simulink subsystem "Tester_subsystem"  (R2023b)
settings: Solver=VariableStepAuto  StartTime=0.0  StopTime=10.0  RelTol=1e-3
settings Model: Creator=nickj  LastModifiedBy=diego

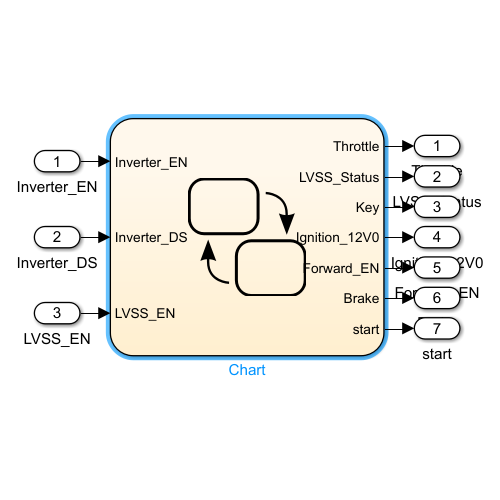
[thumbnail: Simulink's stored preview of the top-level diagram]
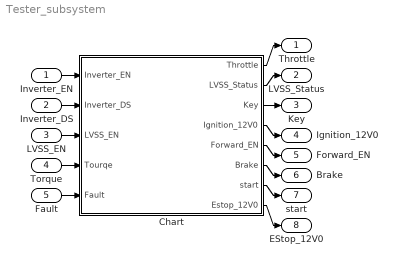
== system Tester_subsystem ==
  Inverter_EN : Inport
  Inverter_DS : Inport  Port=2
  LVSS_EN : Inport  Port=3
  Torque : Inport  Port=4
  Fault : Inport  Port=5
  Chart : Stateflow chart  TreatAsAtomicUnit=on
  Throttle : Outport
  LVSS_Status : Outport  Port=2
  Key : Outport  Port=3
  Ignition_12V0 : Outport  Port=4
  Forward_EN : Outport  Port=5
  Brake : Outport  Port=6
  start : Outport  Port=7
  EStop_12V0 : Outport  Port=8
  wires:
  Chart/3(Key) -> Key/1
  Chart/7(start) -> start/1
  Chart/6(Brake) -> Brake/1
  Chart/1(Throttle) -> Throttle/1
  Inverter_EN/1 -> Chart/1(Inverter_EN)
  Inverter_DS/1 -> Chart/2(Inverter_DS)
  LVSS_EN/1 -> Chart/3(LVSS_EN)
  Chart/4(Ignition_12V0) -> Ignition_12V0/1
  Chart/2(LVSS_Status) -> LVSS_Status/1
  Chart/5(Forward_EN) -> Forward_EN/1
  Torque/1 -> Chart/4(Tourqe)
  Fault/1 -> Chart/5(Fault)
  Chart/8(Estop_12V0) -> EStop_12V0/1

== stateflow chart Tester_subsystem/Chart ==
  state Test_proc
    state Key_Proc
      entry:
      Key = 1;
      Ignition_12V0 = 1;
    state LVSS_Start_Proc
      entry:
      LVSS_Status = 1;
    state Contactor_Closed_Proc
      entry:
      Forward_EN = 1;
      Brake = 1;
      Throttle = 0;
      start = 1;
    state Contactor_Closed_Proc_2
      entry:
      Forward_EN = 1;
      Brake = 1;
      Throttle = 0;
      start = 1;
    state MC_Active_Proc
      entry:
      Forward_EN = 0;
    state MC_Active_Proc1
      entry:
      Ignition_12V0 = 0;
    state LVSS_Shutdown_Proc
      entry:
      LVSS_Status = 0;
    state Off_Proc2
      entry:
      Key = 1;
      Ignition_12V0 = 1;
      LVSS_Status = 1;
    state Init_Proc
      entry:
      Ignition_12V0 = 0;
      LVSS_Status = 0;
    state Off_Proc
      entry:
      Key = 1;
      Ignition_12V0 = 1;
      LVSS_Status = 1;
    state Off_Estop_Proc
      entry:
      Key = 1;
      Ignition_12V0 = 1;
      LVSS_Status = 1;
    state Estop_Proc
      entry:
      Estop_12V0 = 1;
    (default) -> Key_Proc
    Key_Proc -> LVSS_Start_Proc : [LVSS_EN == 1 && Fault == 0]
    Test_proc -> Key_Proc : [LVSS_EN ==0 && Inverter_DS == 1]
    LVSS_Start_Proc -> Contactor_Closed_Proc : [Inverter_DS == 1 && Fault == 0]
    Contactor_Closed_Proc -> MC_Active_Proc : [Inverter_EN == 1 && Tourqe == 0 && Fault == 0]
    MC_Active_Proc -> Contactor_Closed_Proc_2 : [Inverter_EN == 0 && Fault == 0]
    Contactor_Closed_Proc_2 -> MC_Active_Proc1 : [Inverter_EN == 1 && Fault == 0]
    MC_Active_Proc1 -> LVSS_Shutdown_Proc : [Inverter_EN == 0 && Inverter_DS == 1 && Fault == 0]
    LVSS_Shutdown_Proc -> Off_Proc : [LVSS_EN == 0 && Inverter_EN == 0 && Fault == 0]
    Init_Proc -> Off_Proc2 : [LVSS_EN == 0 && Inverter_EN == 0 && Fault == 0]
    Off_Proc -> Init_Proc
    Off_Proc2 -> Estop_Proc : [LVSS_EN == 1]
    Estop_Proc -> Off_Estop_Proc : [LVSS_EN == 0]
  (default) -> Test_proc
  data: Inverter_EN input; Throttle output; LVSS_Status output; Key output; Ignition_12V0 output; Forward_EN output; Brake output; Inverter_DS input; start output; LVSS_EN input; Tourqe input; Fault input; Estop_12V0 output
